simulink model "platooning"  (R2015a)
settings: Solver=ode3  StartTime=0.0  StopTime=8  FixedStep=0.001  RelTol=1e-3
values from neighbouring files (symbols this model uses):
  dt = 1    [Results.m]    (also in dosim2.m = 0.5)
  initF = [-8 0 -0.1]'    [Results.m]    (also in dosim2.m)
  initL = [0 0 0]'    [Results.m]    (also in dosim2.m)
  l = 2    [showpose.m]
  w = 1    [showpose.m]
undefined symbols (not defined in the file or in its folder): f, h, K
settings Model: Creator=yoshi  LastModifiedBy=yoshi

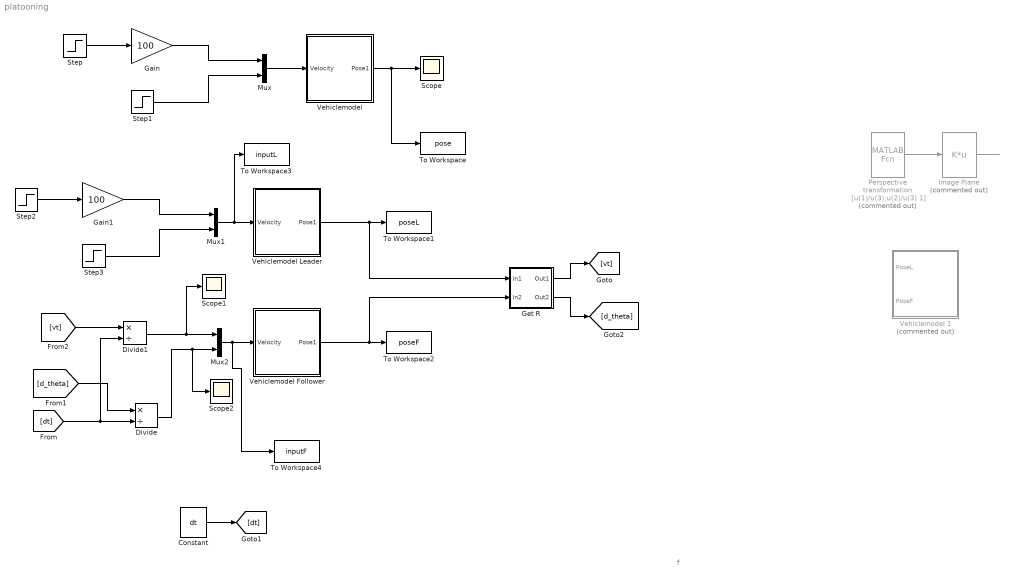
== system platooning ==
  note: f
  Constant : Constant  Value=dt
  Divide : Product  Inputs=*/
  Divide1 : Product  Inputs=*/
  Gain : Gain  Gain=100
  Gain1 : Gain  Gain=100
  Get R : Subsystem
  Image Plane : MATLABFcn  Commented=on  MATLABFcn=K*u  OutputDimensions=[3,1]  Output1D=off
  Mux : Mux  Inputs=2
  Mux1 : Mux  Inputs=2
  Mux2 : Mux  Inputs=2
  Perspective transformation : MATLABFcn  Commented=on  MATLABFcn=[u(1)/u(3);u(2)/u(3) 1]  OutputDimensions=[3,1]  Output1D=off
  Scope : Scope
  Scope1 : Scope
      settings: YMin=-5.5e+11  YMax=3.5e+11
  Scope2 : Scope
      settings: SaveName=ScopeData2
  Step{,1..3} (4 alike) : Step  SampleTime=0
  To Workspace : ToWorkspace  VariableName=pose  SaveFormat=Timeseries  SampleTime=-1
  To Workspace1 : ToWorkspace  VariableName=poseL  SaveFormat=Timeseries  SampleTime=-1
  To Workspace2 : ToWorkspace  VariableName=poseF  SaveFormat=Timeseries  SampleTime=-1
  To Workspace3 : ToWorkspace  VariableName=inputL  SaveFormat=Timeseries  SampleTime=-1
  To Workspace4 : ToWorkspace  VariableName=inputF  SaveFormat=Timeseries  SampleTime=-1
  "Vehiclemodel " : Subsystem
  Vehiclemodel 1 : Subsystem  Commented=on
  Vehiclemodel Follower : Subsystem
  Vehiclemodel Leader : Subsystem
  wires:
  Mux/1 -> "Vehiclemodel "/1(Velocity)
  Gain/1 -> Mux/1
  Step1/1 -> Mux/2
  "Vehiclemodel "/1(Pose1) -> To Workspace/1, Scope/1
  Step/1 -> Gain/1
  Perspective transformation/1 -> Image Plane/1
  Image Plane/1 -> ?
  Mux1/1 -> To Workspace3/1, Vehiclemodel Leader/1(Velocity)
  Gain1/1 -> Mux1/1
  Step3/1 -> Mux1/2
  Step2/1 -> Gain1/1
  Vehiclemodel Leader/1(Pose1) -> Get R/1(In1), To Workspace1/1
  Mux2/1 -> To Workspace4/1, Vehiclemodel Follower/1(Velocity)
  Vehiclemodel Follower/1(Pose1) -> Get R/2(In2), To Workspace2/1
  Get R/1(Out1) -> [vt]
  Divide/1 -> Scope2/1, Mux2/2
  Constant/1 -> [dt]
  [d_theta] -> Divide/1
  [vt] -> Divide1/1
  Divide1/1 -> Scope1/1, Mux2/1
  [dt] -> Divide1/2, Divide/2
  Get R/2(Out2) -> [d_theta]

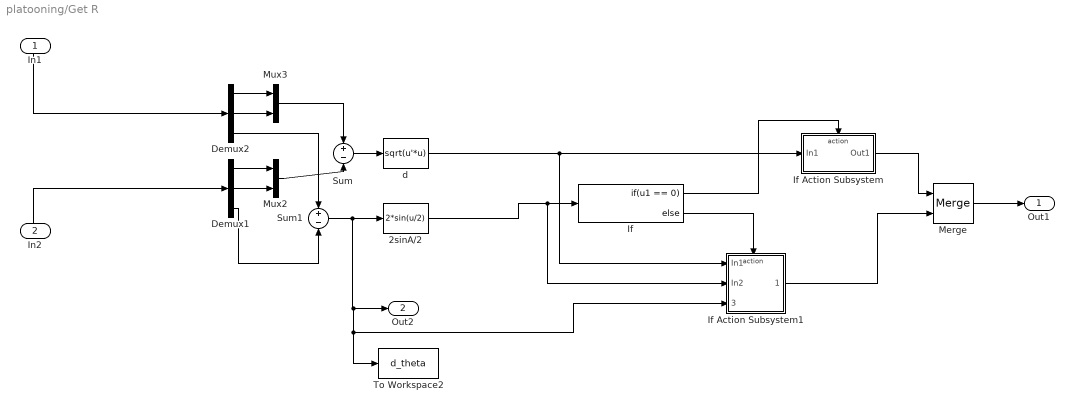
== system platooning/Get R ==
  In1 : Inport
  In2 : Inport  Port=2
  2sinA/2 : MATLABFcn  MATLABFcn=2*sin(u/2)
  Demux1 : Demux  Outputs=3
  Demux2 : Demux  Outputs=3
  If : If  IfExpression=u1 == 0
  If Action Subsystem : Subsystem  TreatAsAtomicUnit=on
  If Action Subsystem1 : Subsystem  TreatAsAtomicUnit=on
  Merge : Merge
  Mux2 : Mux  Inputs=2
  Mux3 : Mux  Inputs=2
  Sum : Sum  Inputs=+|-
  Sum1 : Sum  Inputs=+|-
  To Workspace2 : ToWorkspace  VariableName=d_theta  SaveFormat=Timeseries  SampleTime=-1
  d : MATLABFcn  MATLABFcn=sqrt(u'*u)
  Out1 : Outport
  Out2 : Outport  Port=2
  wires:
  Sum/1 -> d/1
  Mux3/1 -> Sum/1
  Mux2/1 -> Sum/2
  Demux2/3 -> Sum1/1
  Demux1/1 -> Mux2/1
  Demux1/2 -> Mux2/2
  Demux1/3 -> Sum1/2
  In2/1 -> Demux1/1
  In1/1 -> Demux2/1
  2sinA/2/1 -> If Action Subsystem1/2(In2), If/1
  Demux2/1 -> Mux3/1
  Demux2/2 -> Mux3/2
  If/1 -> If Action Subsystem/Action
  d/1 -> If Action Subsystem1/1(In1), If Action Subsystem/1(In1)
  If Action Subsystem/1(Out1) -> Merge/1
  If/2 -> If Action Subsystem1/Action
  If Action Subsystem1/1(Out1) -> Merge/2
  Merge/1 -> Out1/1
  Sum1/1 -> Out2/1, If Action Subsystem1/3("dtheta "), To Workspace2/1, 2sinA/2/1

== system platooning/Vehiclemodel  ==
  Velocity : Inport
  Integrator : Integrator  InitialCondition=[0 0 0]'
  Interpreted MATLAB Function : MATLABFcn  MATLABFcn=[cos(u(3)) 0;sin(u(3)) 0; 0 1];  Output1D=off
  Product : Product  Multiplication=Matrix(*)
  Pose1 : Outport
  wires:
  Product/1 -> Integrator/1
  Velocity/1 -> Product/2
  Integrator/1 -> Interpreted MATLAB Function/1, Pose1/1
  Interpreted MATLAB Function/1 -> Product/1

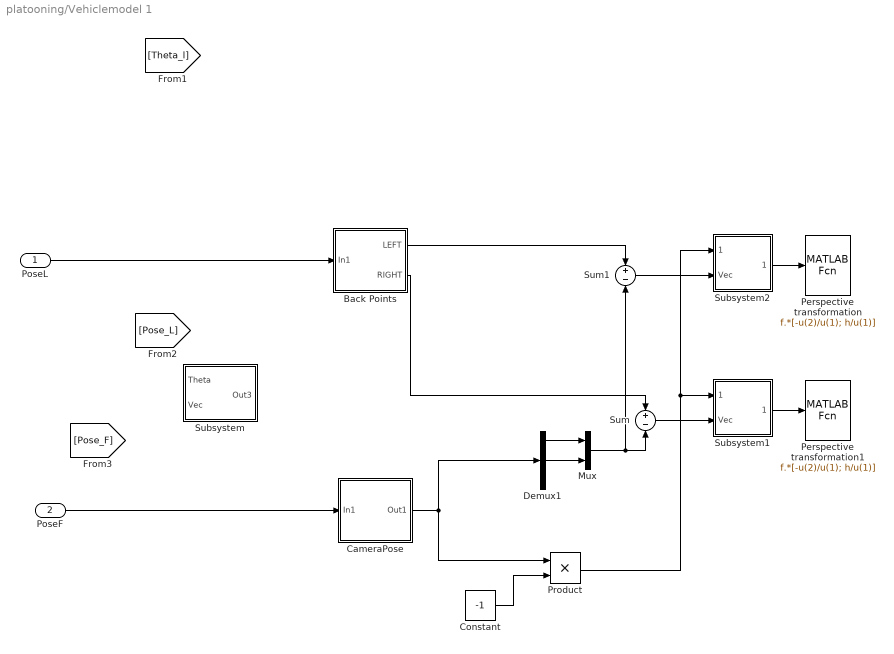
== system platooning/Vehiclemodel 1 ==
  PoseL : Inport
  PoseF : Inport  Port=2
  Back Points : Subsystem
  CameraPose : Subsystem
  Constant : Constant  Value=-1
  Demux1 : Demux  Outputs=3
  Mux : Mux  Inputs=2
  Perspective transformation : MATLABFcn  MATLABFcn=f.*[-u(2)/u(1); h/u(1)]  OutputDimensions=[2,1]  Output1D=off
  Perspective transformation1 : MATLABFcn  MATLABFcn=f.*[-u(2)/u(1); h/u(1)]  OutputDimensions=[2,1]  Output1D=off
  Product : Product
  Subsystem : Subsystem
  Subsystem1 : Subsystem
  Subsystem2 : Subsystem
  Sum : Sum  Inputs=+|-
  Sum1 : Sum  Inputs=+|-
  wires:
  PoseF/1 -> CameraPose/1(In1)
  PoseL/1 -> Back Points/1(In1)
  Back Points/2(RIGHT) -> Sum/1
  CameraPose/1(Out1) -> Demux1/1, Product/1
  Demux1/1 -> Mux/1
  Mux/1 -> Sum/2, Sum1/2
  Demux1/2 -> Mux/2
  Sum/1 -> Subsystem1/2(Vec)
  Constant/1 -> Product/2
  Product/1 -> Subsystem2/1(Theta), Subsystem1/1(Theta)
  Sum1/1 -> Subsystem2/2(Vec)
  Back Points/1("LEFT ") -> Sum1/1
  Subsystem2/1(Out3) -> Perspective transformation/1
  Subsystem1/1(Out3) -> Perspective transformation1/1

== system platooning/Vehiclemodel Follower ==
  Velocity : Inport
  Integrator : Integrator  InitialCondition=initF
  Interpreted MATLAB Function : MATLABFcn  MATLABFcn=[cos(u(3)) 0;sin(u(3)) 0; 0 1];  Output1D=off
  Product : Product  Multiplication=Matrix(*)
  Pose1 : Outport
  wires:
  Product/1 -> Integrator/1
  Velocity/1 -> Product/2
  Integrator/1 -> Interpreted MATLAB Function/1, Pose1/1
  Interpreted MATLAB Function/1 -> Product/1

== system platooning/Vehiclemodel Leader ==
  Velocity : Inport
  Integrator : Integrator  InitialCondition=initL
  Interpreted MATLAB Function : MATLABFcn  MATLABFcn=[cos(u(3)) 0;sin(u(3)) 0; 0 1];  Output1D=off
  Product : Product  Multiplication=Matrix(*)
  Pose1 : Outport
  wires:
  Product/1 -> Integrator/1
  Velocity/1 -> Product/2
  Integrator/1 -> Interpreted MATLAB Function/1, Pose1/1
  Interpreted MATLAB Function/1 -> Product/1

== system platooning/Get R/If Action Subsystem ==
  In1 : Inport
  Action Port : ActionPort  ActionType=then
  Out1 : Outport
  wires:
  In1/1 -> Out1/1

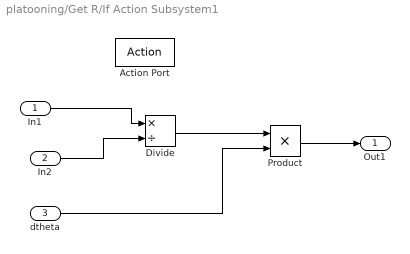
== system platooning/Get R/If Action Subsystem1 ==
  In1 : Inport
  In2 : Inport  Port=2
  "dtheta " : Inport  Port=3
  Action Port : ActionPort  ActionType=else
  Divide : Product  Inputs=*/
  Product : Product
  Out1 : Outport
  wires:
  In1/1 -> Divide/1
  In2/1 -> Divide/2
  Divide/1 -> Product/1
  "dtheta "/1 -> Product/2
  Product/1 -> Out1/1

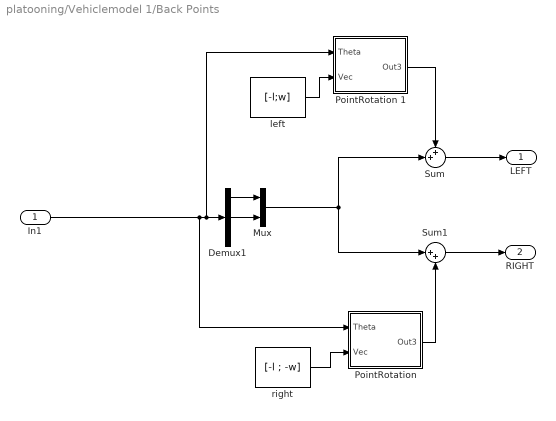
== system platooning/Vehiclemodel 1/Back Points ==
  In1 : Inport
  Demux1 : Demux  Outputs=3
  Mux : Mux  Inputs=2
  "PointRotation " : Subsystem
  PointRotation 1 : Subsystem
  Sum : Sum  Inputs=++|
  Sum1 : Sum  Inputs=|++
  "left " : Constant  Value=[-l;w]  VectorParams1D=off
  right : Constant  Value=[-l ; -w]  VectorParams1D=off
  "LEFT " : Outport
  RIGHT : Outport  Port=2
  wires:
  Sum1/1 -> RIGHT/1
  PointRotation 1/1(Out3) -> Sum/1
  "left "/1 -> PointRotation 1/2(Vec)
  In1/1 -> "PointRotation "/1(Theta), PointRotation 1/1(Theta), Demux1/1
  Sum/1 -> "LEFT "/1
  Demux1/1 -> Mux/1
  Mux/1 -> Sum/2, Sum1/1
  Demux1/2 -> Mux/2
  right/1 -> "PointRotation "/2(Vec)
  "PointRotation "/1(Out3) -> Sum1/2

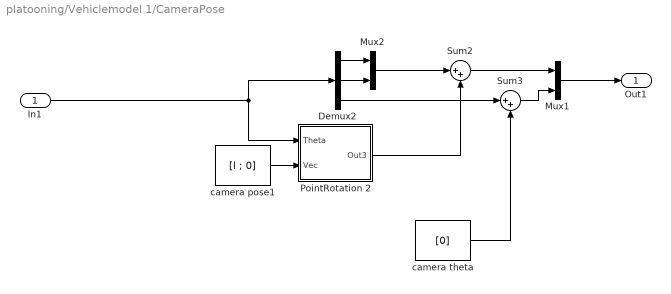
== system platooning/Vehiclemodel 1/CameraPose ==
  In1 : Inport
  Demux2 : Demux  Outputs=3
  Mux1 : Mux  Inputs=2
  Mux2 : Mux  Inputs=2
  PointRotation 2 : Subsystem
  Sum2 : Sum  Inputs=|++
  Sum3 : Sum  Inputs=|++
  camera pose1 : Constant  Value=[l ; 0]  VectorParams1D=off
  camera theta : Constant  Value=[0]  VectorParams1D=off
  Out1 : Outport
  wires:
  Demux2/3 -> Sum3/1
  camera theta/1 -> Sum3/2
  camera pose1/1 -> PointRotation 2/2(Vec)
  Sum2/1 -> Mux1/1
  Mux1/1 -> Out1/1
  Sum3/1 -> Mux1/2
  In1/1 -> PointRotation 2/1(Theta), Demux2/1
  Mux2/1 -> Sum2/1
  Demux2/1 -> Mux2/1
  Demux2/2 -> Mux2/2
  PointRotation 2/1(Out3) -> Sum2/2

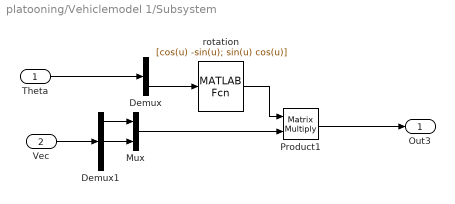
== system platooning/Vehiclemodel 1/Subsystem ==
  Theta : Inport
  Vec : Inport  Port=2
  Demux : Demux  Outputs=3
  Demux1 : Demux  Outputs=3
  Mux : Mux  Inputs=2
  Product1 : Product  Multiplication=Matrix(*)
  rotation : MATLABFcn  MATLABFcn=[cos(u) -sin(u); sin(u) cos(u)]  Output1D=off
  Out3 : Outport
  wires:
  Demux1/1 -> Mux/1
  Demux1/2 -> Mux/2
  Theta/1 -> Demux/1
  rotation/1 -> Product1/1
  Product1/1 -> Out3/1
  Vec/1 -> Demux1/1
  Demux/3 -> rotation/1
  Mux/1 -> Product1/2

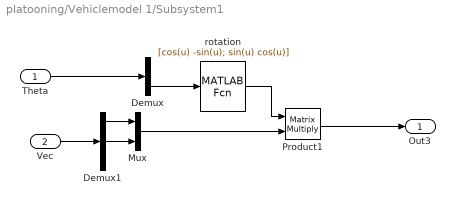
== system platooning/Vehiclemodel 1/Subsystem1 ==
  Theta : Inport
  Vec : Inport  Port=2
  Demux : Demux  Outputs=3
  Demux1 : Demux  Outputs=3
  Mux : Mux  Inputs=2
  Product1 : Product  Multiplication=Matrix(*)
  rotation : MATLABFcn  MATLABFcn=[cos(u) -sin(u); sin(u) cos(u)]  Output1D=off
  Out3 : Outport
  wires:
  Demux1/1 -> Mux/1
  Demux1/2 -> Mux/2
  Theta/1 -> Demux/1
  rotation/1 -> Product1/1
  Product1/1 -> Out3/1
  Vec/1 -> Demux1/1
  Demux/3 -> rotation/1
  Mux/1 -> Product1/2

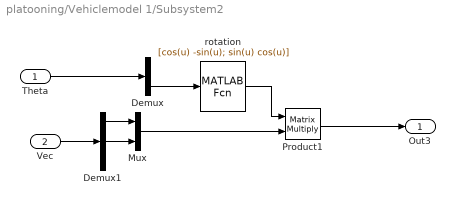
== system platooning/Vehiclemodel 1/Subsystem2 ==
  Theta : Inport
  Vec : Inport  Port=2
  Demux : Demux  Outputs=3
  Demux1 : Demux  Outputs=3
  Mux : Mux  Inputs=2
  Product1 : Product  Multiplication=Matrix(*)
  rotation : MATLABFcn  MATLABFcn=[cos(u) -sin(u); sin(u) cos(u)]  Output1D=off
  Out3 : Outport
  wires:
  Demux1/1 -> Mux/1
  Demux1/2 -> Mux/2
  Theta/1 -> Demux/1
  rotation/1 -> Product1/1
  Product1/1 -> Out3/1
  Vec/1 -> Demux1/1
  Demux/3 -> rotation/1
  Mux/1 -> Product1/2

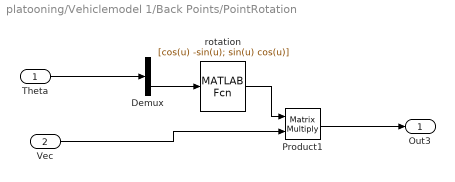
== system platooning/Vehiclemodel 1/Back Points/PointRotation  ==
  Theta : Inport
  Vec : Inport  Port=2
  Demux : Demux  Outputs=3
  Product1 : Product  Multiplication=Matrix(*)
  rotation : MATLABFcn  MATLABFcn=[cos(u) -sin(u); sin(u) cos(u)]  Output1D=off
  Out3 : Outport
  wires:
  Theta/1 -> Demux/1
  rotation/1 -> Product1/1
  Product1/1 -> Out3/1
  Demux/3 -> rotation/1
  Vec/1 -> Product1/2

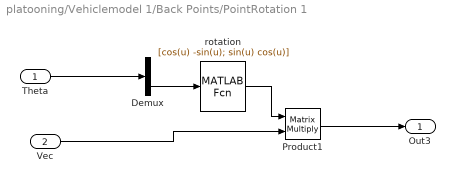
== system platooning/Vehiclemodel 1/Back Points/PointRotation 1 ==
  Theta : Inport
  Vec : Inport  Port=2
  Demux : Demux  Outputs=3
  Product1 : Product  Multiplication=Matrix(*)
  rotation : MATLABFcn  MATLABFcn=[cos(u) -sin(u); sin(u) cos(u)]  Output1D=off
  Out3 : Outport
  wires:
  Theta/1 -> Demux/1
  rotation/1 -> Product1/1
  Product1/1 -> Out3/1
  Demux/3 -> rotation/1
  Vec/1 -> Product1/2

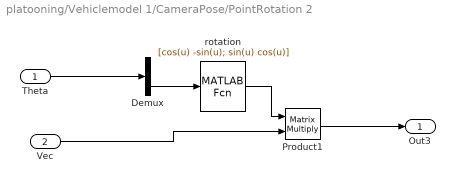
== system platooning/Vehiclemodel 1/CameraPose/PointRotation 2 ==
  Theta : Inport
  Vec : Inport  Port=2
  Demux : Demux  Outputs=3
  Product1 : Product  Multiplication=Matrix(*)
  rotation : MATLABFcn  MATLABFcn=[cos(u) -sin(u); sin(u) cos(u)]  Output1D=off
  Out3 : Outport
  wires:
  Theta/1 -> Demux/1
  rotation/1 -> Product1/1
  Product1/1 -> Out3/1
  Demux/3 -> rotation/1
  Vec/1 -> Product1/2
